simulink model "innerLoopDiscTimeModel_2019b"  (R2019b)
settings: Solver=FixedStepAuto  StartTime=0.0  StopTime=30  FixedStep=0.001  RelTol=1e-3
undefined symbols (not defined in the file or in its folder): D1_den, D1_num, D2_den, D2_num, K2, K3, P_den, P_num, sigAmp, sigDC, sigPeriod, sigPW, T
libraries: simulink x1
settings Model: Creator=adamannosantini  LastModifiedBy=adamannosantini
settings DataIOCC: SaveTime=off
settings DebuggingCC: UnconnectedInputMsg=none  UnconnectedOutputMsg=none  UnconnectedLineMsg=none  SFMachineParentedDataDiag=error

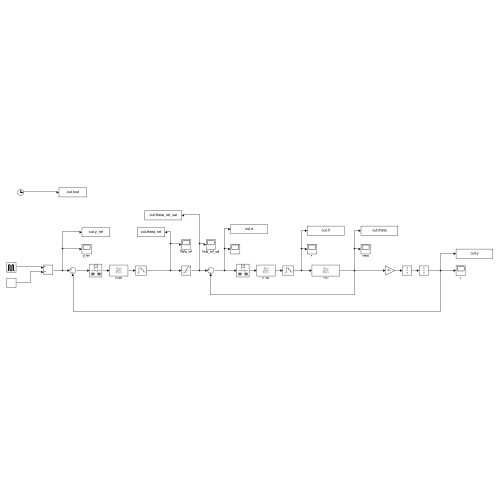
[thumbnail: Simulink's stored preview of the top-level diagram]
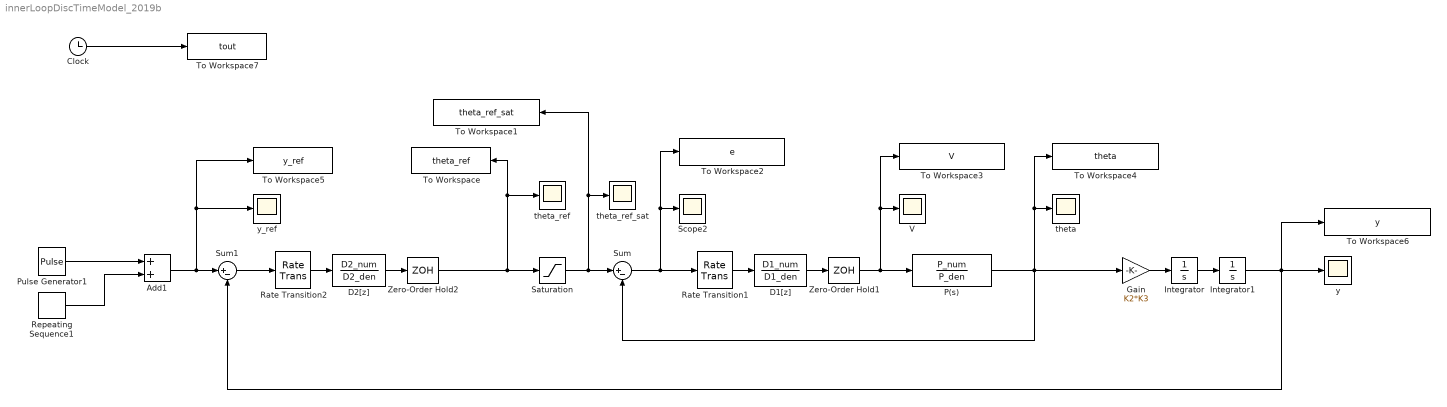
== system innerLoopDiscTimeModel_2019b ==
  Add1 : Sum
  Clock : Clock
  D1[z] : DiscreteTransferFcn  Numerator=D1_num  Denominator=D1_den
  D2[z] : DiscreteTransferFcn  Numerator=D2_num  Denominator=D2_den
  Gain : Gain  Gain=K2*K3
  Integrator : Integrator
  Integrator1 : Integrator
  P(s) : TransferFcn  Numerator=P_num  Denominator=P_den
  Pulse Generator1 : DiscretePulseGenerator  PulseType=Time based  Amplitude=sigAmp  Period=sigPeriod  PulseWidth=sigPW
  Rate Transition1 : RateTransition  OutPortSampleTime=T
  Rate Transition2 : RateTransition  OutPortSampleTime=T
  Repeating Sequence1 : simulink/Sources/Repeating Sequence  rep_seq_t=[0 1]  rep_seq_y=[sigDC sigDC]
  Saturation : Saturate  UpperLimit=pi/4  LowerLimit=-pi/4
  Scope2 : Scope
  Sum : Sum  Inputs=|+-
  Sum1 : Sum  Inputs=|+-
  To Workspace : ToWorkspace  VariableName=theta_ref  SaveFormat=Timeseries  SampleTime=T
  To Workspace1 : ToWorkspace  VariableName=theta_ref_sat  SaveFormat=Timeseries  SampleTime=T
      settings: Save2DSignal=2-D array (concatenate along first dimension)
  To Workspace2 : ToWorkspace  VariableName=e  SaveFormat=Timeseries  SampleTime=T
  To Workspace3 : ToWorkspace  VariableName=V  SaveFormat=Timeseries  SampleTime=T
  To Workspace4 : ToWorkspace  VariableName=theta  SaveFormat=Timeseries  SampleTime=T
  To Workspace5 : ToWorkspace  VariableName=y_ref  SaveFormat=Timeseries  SampleTime=T
  To Workspace6 : ToWorkspace  VariableName=y  SaveFormat=Timeseries  SampleTime=T
  To Workspace7 : ToWorkspace  VariableName=tout  SaveFormat=Timeseries  SampleTime=T
  V : Scope
  Zero-Order Hold1 : ZeroOrderHold  SampleTime=T
  Zero-Order Hold2 : ZeroOrderHold  SampleTime=T
  theta : Scope
  theta_ref : Scope
  theta_ref_sat : Scope
  y : Scope
  y_ref : Scope
  wires:
  P(s)/1 -> Gain/1, To Workspace4/1, theta/1, Sum/2
  Saturation/1 -> To Workspace1/1, theta_ref_sat/1, Sum/1
  Zero-Order Hold2/1 -> To Workspace/1, theta_ref/1, Saturation/1
  Sum/1 -> Rate Transition1/1, To Workspace2/1, Scope2/1
  Zero-Order Hold1/1 -> P(s)/1, To Workspace3/1, V/1
  D1[z]/1 -> Zero-Order Hold1/1
  Rate Transition1/1 -> D1[z]/1
  Integrator/1 -> Integrator1/1
  Gain/1 -> Integrator/1
  Integrator1/1 -> Sum1/2, To Workspace6/1, y/1
  D2[z]/1 -> Zero-Order Hold2/1
  Rate Transition2/1 -> D2[z]/1
  Sum1/1 -> Rate Transition2/1
  Add1/1 -> To Workspace5/1, y_ref/1, Sum1/1
  Clock/1 -> To Workspace7/1
  Pulse Generator1/1 -> Add1/1
  Repeating Sequence1/1 -> Add1/2
